simulink model "model11"  (R2013b)
settings: Solver=ode45  StartTime=0.0  StopTime=10.0  RelTol=1e-3
settings Model: Creator=Axel  LastModifiedBy=Axel
settings OptimizationCC: InlineParams=on
settings DebuggingCC: StateNameClashWarn=warning

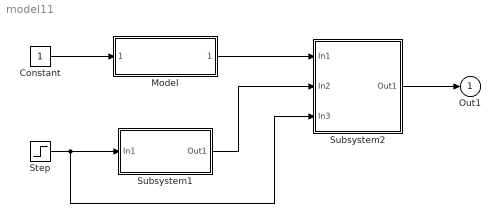
== system model11 ==
  Constant : Constant
  Model : ModelReference  ModelNameDialog=model3  ModelReferenceVersion=1.4  CopyOfModelName=model3  DefaultDataLogging=on
  Step : Step
  Subsystem1 : Subsystem
  Subsystem2 : Subsystem
  Out1 : Outport
  wires:
  Constant/1 -> Model/1
  Step/1 -> Subsystem2/3(In3), Subsystem1/1(In1)
  Model/1 -> Subsystem2/1(In1)
  Subsystem1/1(Out1) -> Subsystem2/2(In2)
  Subsystem2/1(Out1) -> Out1/1

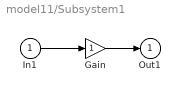
== system model11/Subsystem1 ==
  In1 : Inport
  Gain : Gain  SaturateOnIntegerOverflow=on  OutDataTypeStr=Inherit: Same as input  ParamDataTypeStr=Inherit: Same as input
  Out1 : Outport
  wires:
  In1/1 -> Gain/1
  Gain/1 -> Out1/1

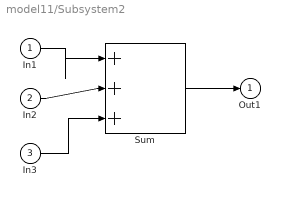
== system model11/Subsystem2 ==
  In1 : Inport
  In2 : Inport  Port=2
  In3 : Inport  Port=3
  Sum : Sum  Inputs=|+++  SaturateOnIntegerOverflow=on  InputSameDT=on  OutDataTypeStr=Inherit: Same as first input
  Out1 : Outport
  wires:
  In1/1 -> Sum/1
  In2/1 -> Sum/2
  In3/1 -> Sum/3
  Sum/1 -> Out1/1
